simulink model "SistemaCAS_v8"  (R2014a)
settings: Solver=ode3  StartTime=0.0  StopTime=500  RelTol=1e-3
settings Model: Creator=andre  LastModifiedBy=andre

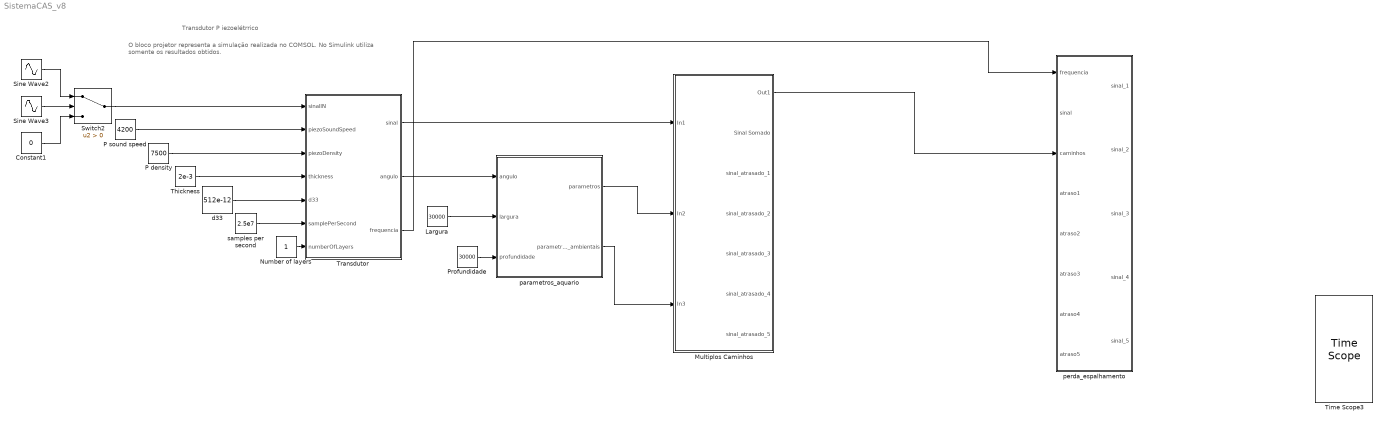
== system SistemaCAS_v8 ==
  note: O bloco projetor representa a simulação realizada no COMSOL. No Simulink utiliza somente os resultados obtidos.
  note: Transdutor P iezoelétrrico
  Constant1 : Constant  Value=0
  Largura : Constant  Value=30000
  Multiplos Caminhos : Subsystem
  Number of layers : Constant
  P density : Constant  Value=7500
  P sound speed : Constant  Value=4200
  Profundidade : Constant  Value=30000
  Sine Wave2 : Sin  Frequency=5  SampleTime=0
  Sine Wave3 : Sin  SampleTime=0
  Switch2 : Switch  Criteria=u2 > Threshold
  Thickness : Constant  Value=2e-3
  Time Scope3 : TimeScope  NumInputPorts=6  DefaultConfigurationName=spbscopes.TimeScopeBlockCfg
  Transdutor : MATLAB Function  TreatAsAtomicUnit=on
  d33 : Constant  Value=512e-12
  parametros_aquario : MATLAB Function  TreatAsAtomicUnit=on
  perda_espalhamento : MATLAB Function  TreatAsAtomicUnit=on
  samples per second : Constant  Value=2.5e7
  wires:
  Largura/1 -> parametros_aquario/2(largura)
  Profundidade/1 -> parametros_aquario/3(profundidade)
  d33/1 -> Transdutor/5(d33)
  samples per second/1 -> Transdutor/6(samplePerSecond)
  Number of layers/1 -> Transdutor/7(numberOfLayers)
  P sound speed/1 -> Transdutor/2(piezoSoundSpeed)
  P density/1 -> Transdutor/3(piezoDensity)
  Thickness/1 -> Transdutor/4(thickness)
  Transdutor/2(angulo) -> parametros_aquario/1(angulo)
  Sine Wave2/1 -> Switch2/1
  Sine Wave3/1 -> Switch2/2
  Constant1/1 -> Switch2/3
  Switch2/1 -> Transdutor/1(sinalIN)
  Transdutor/1(sinal) -> Multiplos Caminhos/1(In1)
  parametros_aquario/1(parametros) -> Multiplos Caminhos/2(In2)
  parametros_aquario/2(parametros_ambientais) -> Multiplos Caminhos/3(In3)
  Multiplos Caminhos/1(Out1) -> perda_espalhamento/3(caminhos)
  Transdutor/3(frequencia) -> perda_espalhamento/1(frequencia)

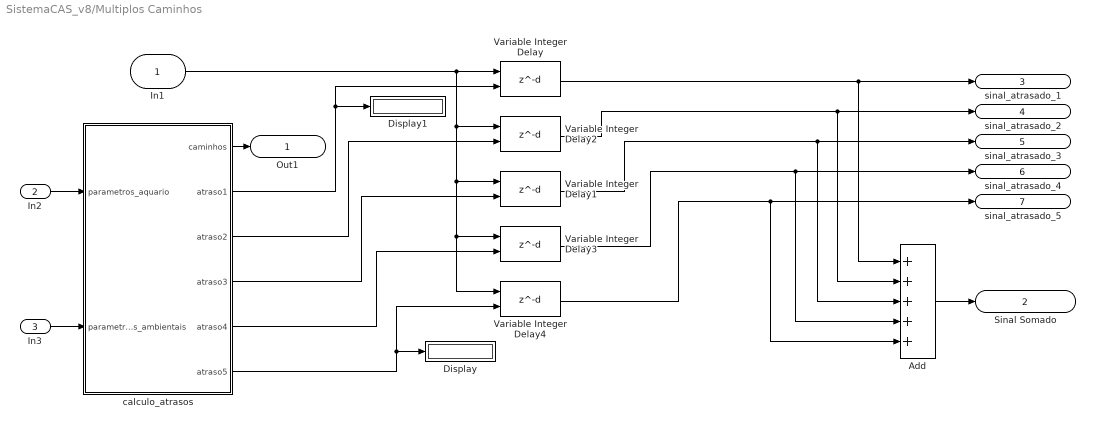
== system SistemaCAS_v8/Multiplos Caminhos ==
  In1 : Inport
  In2 : Inport  Port=2
  In3 : Inport  Port=3
  Add : Sum  Inputs=+++++
  Display : Display
  Display1 : Display
  Variable Integer Delay{,1..4} (5 alike) : Delay  DelayLengthSource=Input port
      settings: InputPortMap=u0,p1
  calculo_atrasos : MATLAB Function  TreatAsAtomicUnit=on
  Out1 : Outport
  Sinal Somado : Outport  Port=2
  sinal_atrasado_1 : Outport  Port=3
  sinal_atrasado_2 : Outport  Port=4
  sinal_atrasado_3 : Outport  Port=5
  sinal_atrasado_4 : Outport  Port=6
  sinal_atrasado_5 : Outport  Port=7
  wires:
  calculo_atrasos/5(atraso4) -> Variable Integer Delay3/2
  calculo_atrasos/4(atraso3) -> Variable Integer Delay1/2
  Add/1 -> Sinal Somado/1
  In2/1 -> calculo_atrasos/1(parametros_aquario)
  In3/1 -> calculo_atrasos/2(parametros_ambientais)
  Variable Integer Delay4/1 -> Add/5, sinal_atrasado_5/1
  Variable Integer Delay3/1 -> Add/4, sinal_atrasado_4/1
  Variable Integer Delay2/1 -> Add/2, sinal_atrasado_2/1
  calculo_atrasos/1(caminhos) -> Out1/1
  Variable Integer Delay1/1 -> Add/3, sinal_atrasado_3/1
  Variable Integer Delay/1 -> Add/1, sinal_atrasado_1/1
  In1/1 -> Variable Integer Delay4/1, Variable Integer Delay3/1, Variable Integer Delay1/1, Variable Integer Delay2/1, Variable Integer Delay/1
  calculo_atrasos/3(atraso2) -> Variable Integer Delay2/2
  calculo_atrasos/2(atraso1) -> Display1/1, Variable Integer Delay/2
  calculo_atrasos/6(atraso5) -> Variable Integer Delay4/2, Display/1

== matlab function SistemaCAS_v8/parametros_aquario ==
  data: angulo input; largura input; profundidade input; parametros output; parametros_ambientais output
function [parametros,parametros_ambientais] = parametros_aquario(angulo,largura,profundidade)
% consideraçoes para os parâmetros do aquário
% 1. emissor e receptor estão alinhados ( largura(x) e profundidade(z)
% iguais, só muda o comprimento (y)
% 2. o comprimento do aquario (L) é ideal para acontecer uma reflexão completa
% com o angulo de diretividade (que é o maior angulo possível do lóbulo 
% principal utilizando o transdutor piezoeletrico escolhido)
% 3. para facilitar os cálculos de do comprimento ideal, utilizamos largura
% igual profundidade (D = W)

% considerações sobre a simulação
% 1. serão considerados somente os caminhos do angulo de diretividade e o
% caminho direto (5 caminhos: um direto, dois que refletem nas laterais, e
% dois que refletem na superfície e o fundo
% 2. a reflexão será considerada reflexão completa com um eco (sem perdas 
% de energia ou refraçao)

%-------------------------------------------------------------------------
%Parâmetros do Aquário definidos anteriormente
%-------------------------------------------------------------------------
w = largura;                  % largura (eixo x)
d = profundidade;             % profundidade do aquário (eixo z) 
l = w/sin(angulo/2);      % comprimento do aquário calculado utilizando o angulo de diretividade (eixo y)
% l(éle) é a distancia ideal para acontecer uma reflexão completa
parametros = [w,l,d];


%-------------------------------------------------------------------------
% Valores dos parâmetros do meio subaquático 
%-------------------------------------------------------------------------
T = 32;                 % Temperatura (°C)
S = 1;                  % Salinidade (ppt)
pH = 7.2;               % acidêz da água - pH (potencial hidrogeniônico)
parametros_ambientais = [T, S, pH];

== matlab function SistemaCAS_v8/Multiplos Caminhos/calculo_atrasos ==
  data: caminhos output; atraso1 output; atraso2 output; atraso3 output; atraso4 output; atraso5 output; parametros_aquario input; parametros_ambientais input
function [caminhos,atraso1,atraso2,atraso3,atraso4,atraso5] = calculo_atrasos(parametros_aquario,parametros_ambientais)
%Definir as distâncias de cada caminho
%Atrasar o sinal de cada caminho
%Enviar a distância e o sinal de cada caminho ()

w = parametros_aquario(1);
l = parametros_aquario(2);
d = parametros_aquario(3);

T = parametros_ambientais(1);
S = parametros_ambientais(2);
pH = parametros_ambientais(3);

%%%%%%  Bloco multipath  %%%%%%

%-------------------------------------------------------------------------
%Definindo as distâncias de cada caminho do multipath
%-------------------------------------------------------------------------
% caminho_1 = caminho refletido na superfície
% caminho_2 = caminho refletido na lateral de trás
% caminho_3 = caminho direto
% caminho_4 = caminho refletido na lateral da frente
% caminho_5 = caminho refletido no fundo
caminhos = [0 0 0 0 0];
caminhos(1) = sqrt(d^2 + l^2);
caminhos(2) = sqrt(w^2 + l^2);
caminhos(3) = l;
caminhos(4) = caminhos(2);
caminhos(5) = caminhos(1);

%-------------------------------------------------------------------------
%Definindo a profundidade média para cada caminho
%-------------------------------------------------------------------------
D = [0 0 0 0 0];
D(1) = mean([d/2,0]);
D(2) = d/2;
D(3) = d/2;
D(4) = d/2;
D(5) = mean([d,d/2]);

%-------------------------------------------------------------------------
%Velocidade do som na água (m/s)
%-------------------------------------------------------------------------
C = [0 0 0 0 0];
for i = 1:5 %5 caminhos
    c = 1448.96 + 4.591*T - 5.304*(10^(-2))*(T^(2))...
        + 2.374*(10^(-4))*(T^(3)) + 1.340*(S-35) + 1.630*(10^(-2))*D(i)...
        + 1.675*(10^(-7))*(D(i)^(2)) - 1.025*(10^(-2))*T*(S-35)...
        - 7.139*(10^(-13))*T*(D(i)^(3));
    
    %Conversão de (m/s) para (cm/s)
    C(i)=c*100;
end

%-------------------------------------------------------------------------
% Definindo os atrasos de cada caminho do multipath através da equação de
% velocidade de propagação do som na água
%-------------------------------------------------------------------------

% atraso é o tempo que o caminho leva

atraso1 = 100*D(1)/C(1);
atraso2 = 100*D(2)/C(2);
atraso3 = 100*D(3)/C(3); % caminho direto não tem atraso
atraso4 = 100*D(4)/C(4);
atraso5 = 100*D(5)/C(5);

== matlab function SistemaCAS_v8/perda_espalhamento ==
  data: frequencia input; sinal input; caminhos input; sinal_1 output; sinal_2 output; sinal_3 output; sinal_4 output; sinal_5 output; atraso1 input; atraso2 input; atraso3 input; atraso4 input; atraso5 input
function [sinal_1,sinal_2,sinal_3,sinal_4, sinal_5]  = perda_espalhamento(frequencia,sinal,caminhos,atraso1,atraso2,atraso3,atraso4,atraso5)


%Speed of sound (m/s)
cmetro = 1448.96 + 4.591*T - 5.304*(10^(-2))*(T^(2)) +...
    + 2.374*(10^(-4))*(T^(3))...
    + 1.340*(S-35) + 1.630*(10^(-2))*D + 1.675*(10^(-7))*(D^(2)) +...
    - 1.025*(10^(-2))*T*(S-35) - 7.139*(10^(-13))*T*(D^(3));

%Conversion from m/s to cm/s
c=cmetro*100;

%Calculation of wavelength
lambda = c/(f*1000);

%Calculation of the transducer diameter
angulo = 0;
d = 2*r;
de = (pi*rr^2);

== matlab function SistemaCAS_v8/Transdutor ==
  data: sinalIN input; sinal output; piezoSoundSpeed input; piezoDensity input; thickness input; d33 input; samplePerSecond input; numberOfLayers input; angulo output; frequencia output
function [sinal, angulo, frequencia] = projetor(sinalIN, piezoSoundSpeed, piezoDensity, thickness, d33, samplePerSecond, numberOfLayers)


%-------------------------------------------------------------------------
% Sinal 
%-------------------------------------------------------------------------
sinal=sinalIN;

%-------------------------------------------------------------------------
% Ângulo de diretividade do transdutor calculado no COMSOL (rad)
%-------------------------------------------------------------------------
angulo = pi/3;            % (ex.: 60º = pi/3 rad)

%-------------------------------------------------------------------------
% Frequência do Sinal (kHz)
%-------------------------------------------------------------------------
frequencia = 1:2:2000;
